simulink model "sldv_deadpath"  (R2015b)
settings: Solver=FixedStepDiscrete  SolverMode=SingleTasking  StartTime=0.0  StopTime=10.0  RelTol=1e-3
Description:
  | Model Coverage Test Generation
settings Model: Creator=The MathWorks Inc.  LastModifiedBy=amatsumo
settings DataIOCC: SaveFormat=Array  SignalLoggingSaveFormat=ModelDataLogs  SaveOutput=off  SignalLogging=off  SaveTime=off
settings OptimizationCC: BlockReduction=off  ConditionallyExecuteInputs=off  DefaultParameterBehavior=Inlined  ExpressionDepthLimit=2147483647  InitFltsAndDblsToZero=on  EfficientMapNaN2IntZero=off
settings DebuggingCC: AlgebraicLoopMsg=error  SaveWithParameterizedLinksMsg=none  UnderspecifiedInitializationDetection=Classic  MergeDetectMultiDrivingBlocksExec=none  SignalResolutionControl=TryResolveAllWithWarning  SolverPrmCheckMsg=warning  SingleTaskRateTransMsg=error  FcnCallInpInsideContextMsg=UseLocalSettings  StateNameClashWarn=warning
settings HardwareCC: ProdBitPerPointer=32  ProdLargestAtomicFloat=None  ProdIntDivRoundTo=Undefined  ProdEndianess=Unspecified  ProdWordSize=32  ProdHWDeviceType=ASIC/FPGA->ASIC/FPGA  ProdEqTarget=off
settings SFSimCC: SimParseCustomCode=off
settings GRTTargetCC: TargetFcnLib=ansi_tfl_tmw.mat  GeneratePreprocessorConditionals=Disable all  CombineOutputUpdateFcns=off  GRTInterface=on
settings ConfigComp: RecordCoverage=on  CovModelRefEnable=Off  CovSFcnEnable=off  DVMaxProcessTime=60  DVDisplayUnsatisfiableObjectives=on  DVAutomaticStubbing=off  DVMakeOutputFilesUnique=off  DVParameters=on  DVModelCoverageObjectives=MCDC  DVMaxTestCaseSteps=500  DVTestSuiteOptimization=CombinedObjectives  DVAssertions=EnableAll  DVProofAssumptions=EnableAll  DVDetectActiveLogic=on  DVProvingStrategy=FindViolation  DVSaveHarnessModel=on  DVModelReferenceHarness=on  DVSaveReport=on  DVActiveTab=3

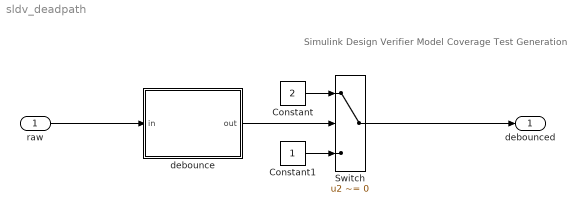
== system sldv_deadpath ==
  note: Simulink Design Verifier
      | Model Coverage Test Generation
  raw : Inport  OutDataTypeStr=uint8
  Constant : Constant  Value=2  OutDataTypeStr=uint8
  Constant1 : Constant  OutDataTypeStr=uint8
  Switch : Switch  Criteria=u2 ~= 0
  debounce : Stateflow chart  TreatAsAtomicUnit=on
  debounced : Outport  OutDataTypeStr=uint8
  wires:
  raw/1 -> debounce/1(in)
  debounce/1(out) -> Switch/2
  Switch/1 -> debounced/1
  Constant/1 -> Switch/1
  Constant1/1 -> Switch/3

== stateflow chart sldv_deadpath/debounce ==
  settings: updateMethod=DISCRETE  sampleTime=0.01  stateMachineType=MOORE_MACHINE  executeAtInitialization=1  initializeOutput=1
  state Wait
    state To_on
    state To_off
  state Off
    out = 0;
  state On
    out = 1;
  Off -> On [order 2] : [in < 0]
  (default) -> Off
  Off -> To_on [order 1] : [in==1]
  To_on -> On [order 2] : [after(5,tick)]
  To_on -> Off [order 1] : [in==0]
  To_off -> Off [order 2] : [after(5,tick)]
  On -> To_off : [in==0]
  To_off -> On [order 1] : [in==1]
  data: in input uint8; out output uint8
